simulink model "OFDM_Transceiver"  (R2013b)
settings: Solver=ode45  StartTime=0.0  StopTime=10.0  RelTol=1e-3
undefined symbols (not defined in the file or in its folder): A, N, xlipgetpartsetting
libraries: xbsIndex_r4 x35, commchan3 x2, commsink2 x2, commrandsrc2 x1, JTAGRuntimeCosim_r4 x1
settings Model: Creator=Lenovo  LastModifiedBy=Lenovo
settings OptimizationCC: ExpressionDepthLimit=2147483647
settings DebuggingCC: StateNameClashWarn=warning

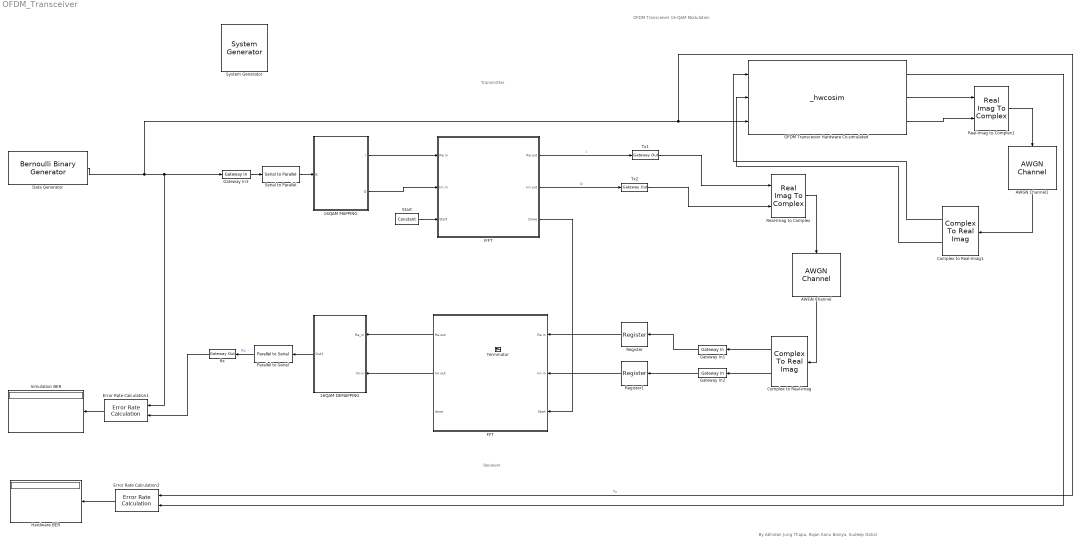
== system OFDM_Transceiver ==
  note: Transmitter
  note: Receiver
  note: OFDM Transceiver 16-QAM Modulation
  note: By Abhidan Jung Thapa, Rajan Kanu Baniya, Sudeep Dahal
  " System Generator" : xbsIndex_r4/ System Generator  Tag=genX  xilinxfamily=spartan3e  part=xc3s500e  speed=-4  package=fg320  synthesis_tool=XST  clock_wrapper=Clock Enables  directory=./netlist  proj_type=Project Navigator  Synth_file=XST Defaults  Impl_file=ISE Defaults  testbench=off  simulink_period=1  sysclk_period=20  dcm_input_clock_period=100  incr_netlist=off  trim_vbits=Everywhere in SubSystem  dbl_ovrd=According to Block Masks  core_generation=According to Block Masks  run_coregen=off  deprecated_control=off  eval_field=0  block_type=sysgen
      settings: block_version=10.1.3
  "16QAM DEMAPPING " : Subsystem
      mask Display: patch([0.363636 0.290909 0.4 0.290909 0.363636 0.490909 0.527273 0.563636 0.690909 0.581818 0.472727 0.4 0.509091 0.4 0.472727 0.581818 0.690909 0.563636 0.527273 0.490909 0.363636 ],[0.115385 0.269231 0.5 0.730769 0.884615 0.884615 0.807692 0.884615 0.884615 0.653846 0.884615 0.730769 0.5 0.269231 0.115385 0.346154 0.115385 0.115385 0.192308 0.115385 0.115385 ],[0.98 0.96 0.92]);
  16QAM MAPPING : Subsystem
      mask Display: patch([0.363636 0.290909 0.4 0.290909 0.363636 0.490909 0.527273 0.563636 0.690909 0.581818 0.472727 0.4 0.509091 0.4 0.472727 0.581818 0.690909 0.563636 0.527273 0.490909 0.363636 ],[0.115385 0.269231 0.5 0.730769 0.884615 0.884615 0.807692 0.884615 0.884615 0.653846 0.884615 0.730769 0.5 0.269231 0.115385 0.346154 0.115385 0.115385 0.192308 0.115385 0.115385 ],[0.98 0.96 0.92]);
  AWGN Channel : commchan3/AWGN Channel  InputProcessing=Inherited (this choice will be removed - see release notes)  seed=67  noiseMode="Signal to noise ratio  (SNR)"  EbNodB=10  EsNodB=40  SNRdB=20  bitsPerSym=2  Ps=1  Tsym=4e-6/80  variance=1
  AWGN Channel1 : commchan3/AWGN Channel  InputProcessing=Inherited (this choice will be removed - see release notes)  seed=67  noiseMode="Signal to noise ratio  (SNR)"  EbNodB=10  EsNodB=40  SNRdB=20  bitsPerSym=2  Ps=1  Tsym=4e-6/80  variance=1
  Complex to Real-Imag : ComplexToRealImag
  Complex to Real-Imag1 : ComplexToRealImag
  Data Generator : commrandsrc2/Bernoulli Binary Generator  P=0.5  seed=61  Ts=1  frameBased=off  sampPerFrame=1  orient=off  outDataType=double
  Error Rate Calculation1 : commsink2/Error Rate Calculation  N=1672  st_delay=700  cp_mode=Entire frame  subframe=[]  PMode=Port  WsName=ErrorVec  RsMode2=off  stop=off  numErr=100  maxBits=1e6
  Error Rate Calculation2 : commsink2/Error Rate Calculation  N=1672  st_delay=700  cp_mode=Entire frame  subframe=[]  PMode=Port  WsName=ErrorVec  RsMode2=off  stop=off  numErr=100  maxBits=1e6
  FFT : Subsystem
      mask Display: patch([0.363636 0.290909 0.4 0.290909 0.363636 0.490909 0.527273 0.563636 0.690909 0.581818 0.472727 0.4 0.509091 0.4 0.472727 0.581818 0.690909 0.563636 0.527273 0.490909 0.363636 ],[0.115385 0.269231 0.5 0.730769 0.884615 0.884615 0.807692 0.884615 0.884615 0.653846 0.884615 0.730769 0.5 0.269231 0.115385 0.346154 0.115385 0.115385 0.192308 0.115385 0.115385 ],[0.98 0.96 0.92]);
  Gateway In1 : xbsIndex_r4/Gateway In  gui_display_data_type=Fixed-point  arith_type="Signed  (2's comp)"  n_bits=16  bin_pt=15  preci_type=Single  exp_width=8  frac_width=24  quantization="Round  (unbiased: +/- Inf)"  overflow=Saturate  period=4  dbl_ovrd=off  timing_constraint=None  locs_specified=off  LOCs={}  UseAsADC=off  ADCChannel='1'  inherit_from_input=off  hdl_port=on  block_type=gatewayin
  Gateway In2 : xbsIndex_r4/Gateway In  gui_display_data_type=Fixed-point  arith_type="Signed  (2's comp)"  n_bits=16  bin_pt=15  preci_type=Single  exp_width=8  frac_width=24  quantization="Round  (unbiased: +/- Inf)"  overflow=Saturate  period=4  dbl_ovrd=off  timing_constraint=None  locs_specified=off  LOCs={}  UseAsADC=off  ADCChannel='1'  inherit_from_input=off  hdl_port=on  block_type=gatewayin
  Gateway In3 : xbsIndex_r4/Gateway In  gui_display_data_type=Fixed-point  arith_type=Unsigned  n_bits=1  bin_pt=0  preci_type=Single  exp_width=8  frac_width=24  quantization="Round  (unbiased: +/- Inf)"  overflow=Saturate  period=1  dbl_ovrd=off  timing_constraint=None  locs_specified=off  LOCs={}  UseAsADC=off  ADCChannel='1'  inherit_from_input=off  hdl_port=on  block_type=gatewayin
  Hardware BER : Display
  IFFT : Subsystem
      mask Display: patch([0.363636 0.290909 0.4 0.290909 0.363636 0.490909 0.527273 0.563636 0.690909 0.581818 0.472727 0.4 0.509091 0.4 0.472727 0.581818 0.690909 0.563636 0.527273 0.490909 0.363636 ],[0.115385 0.269231 0.5 0.730769 0.884615 0.884615 0.807692 0.884615 0.884615 0.653846 0.884615 0.730769 0.5 0.269231 0.115385 0.346154 0.115385 0.115385 0.192308 0.115385 0.115385 ],[0.98 0.96 0.92]);
  "OFDM Transceiver Hardware Co-simulated " : JTAGRuntimeCosim_r4/_hwcosim  clkSrc=Single Stepped  hasCombinationalPath=on  bitfileName=E:\FPGA\FinalYearProject\netlist\ofdm_final_october31_cw.bit  skipConfig=off  cable=Auto Detect  speed=N/A  cablePort=N/A  cableLocation=Local  shareCable=off  enable_codebug=on  design_xtable=|  engineDll=JTAGCosimEngine.dll  cableWaitTime=10  bscanPos=1  IRLengths=[6,8,8]  useWaitBox=1  hasBufgmux=on  Scheme=Cosim  useCmdProc=1  hasProc=0  useImpact=0  printLogFile=0  block_type=jtagcosim
      | {
      |   'clkWrapper' => 'ofdm_final_october31_cw',
      |   'clocksGcd' => undef,
      |   'device' => 'xc3s500e-4fg320',
      |   'ports' => {
      |     'gateway_in1' => {
      |       'bd_port_index' => 0,
      |       'direction' => 'in',
      |       'icon_text' => 'Gateway In1',
      |       'period' => 4,
      |       'sim_pause_trigger' => false,
      |       'type' => 'Fix_16_15',
      |       'width' => 16,
      |     },
      |     'gateway_in2' => {
      |       'bd_port_index' => 1,
      |       'direction' => 'in',
      |       'icon_text' => 'Gateway In2',
      |       'period' => 4,
      |       'sim_pause_trigger' => false,
      |       'type' => 'Fix_16_15',
      |       'width' => 16,
      |     },
      |     'gateway_in3' => {
      |       'bd_port_index' => 2,
      |       'direction' => 'in',
      |       'icon_text' => 'Gateway In3',
      |       'period' => 1,
      |       'sim_pause_trigger' => false,
      |       'type' => 'UFix_1_0',
      |       'width' => 1,
      |     },
      |     'rx' => {
      |       'bd_port_index' => 0,
      |       'direction' => 'out',
      |       'icon_text' => 'Rx',
      |       'period' => 1,
      |       'sim_pause_trigger' => false,
      |       'type' => 'UFix_1_0',
      |       'width' => 1,
      |     },
      |     'tx1' => {
      |       'bd_port_index' => 1,
      |       'direction' => 'out',
      |       'icon_text' => 'Tx1',
      |       'period' => 4,
      |       'sim_pause_trigger' => false,
      |       'type' => 'Fix_16_15',
      |       'width' => 16,
      |     },
      |     'tx2' => {
      |       'bd_port_index' => 2,
      |       'direction' => 'out',
      |       'icon_text' => 'Tx2',
      |       'period' => 4,
      |       'sim_pause_trigger' => false,
      |       'type' => 'Fix_16_15',
      |       'width' => 16,
      |     },
      |   },
      |   'shared_memories' => {},
      | }
  Parallel to Serial : xbsIndex_r4/Parallel to Serial  output_order=Least Significant Word First  arith_type=Unsigned  output_bits=1  bin_pt=0  rst=off  en=off  latency=0  dbl_ovrd=off  block_type=p2s
      settings: infoedit=Each sample presented at the input becomes several samples presented serially at the output.  xl_area=[4 5 0 4 0 0 0]  block_version=10.1.3
  Real-Imag to Complex : RealImagToComplex
  Real-Imag to Complex1 : RealImagToComplex
  Register : xbsIndex_r4/Register  init=0  rst=off  en=off  dbl_ovrd=off  block_type=register
  Register1 : xbsIndex_r4/Register  init=0  rst=off  en=off  dbl_ovrd=off  block_type=register
  Rx : xbsIndex_r4/Gateway Out  inherit_from_input=off  hdl_port=on  timing_constraint=None  locs_specified=off  LOCs={}  UseAsDAC=off  DACChannel='1'  block_type=gatewayout
      settings: infoedit="Gateway out block.  Converts Xilinx fixed point inputs into ouputs of type Simulink integer, double, or fixed point.<br><br>Hardware notes:  In hardware these blocks become top level output ports or are discarded, depending on how they are configured."  block_version=10.1.3
  Serial to Parallel : xbsIndex_r4/Serial to Parallel  input_order=Least Significant Word First  arith_type=Unsigned  output_bits=4  bin_pt=0  rst=off  en=off  latency=1  dbl_ovrd=off  block_type=s2p
      settings: infoedit=Groups of samples presented serially at the input become single samples presented at the output.  xl_area=[4 8 0 1 0 0 0]  block_version=10.1.3
  Simulation BER : Display
  Start : xbsIndex_r4/Constant  const=1  gui_display_data_type=Fixed-point  arith_type=Boolean  n_bits=16  bin_pt=14  preci_type=Single  exp_width=8  frac_width=24  explicit_period=off  period=1  equ=P=C  opselect=C  inp2=PCIN>>17  opr=+  inp1=P  carry=CIN  dbl_ovrd=off  block_type=constant
  Terminator : Terminator
  Tx1 : xbsIndex_r4/Gateway Out  inherit_from_input=off  hdl_port=on  timing_constraint=None  locs_specified=off  LOCs={}  UseAsDAC=off  DACChannel='1'  block_type=gatewayout
      settings: block_version=10.1.3
  Tx2 : xbsIndex_r4/Gateway Out  inherit_from_input=off  hdl_port=on  timing_constraint=None  locs_specified=off  LOCs={}  UseAsDAC=off  DACChannel='1'  block_type=gatewayout
      settings: block_version=10.1.3
  wires:
  Error Rate Calculation1/1 -> Simulation BER/1
  IFFT/3(Done) -> FFT/3(Start)
  Parallel to Serial/1 -> Rx/1  "Rx"
  Serial to Parallel/1 -> 16QAM MAPPING/1(B)
  Start/1 -> IFFT/3(Start)
  16QAM MAPPING/2(Q) -> IFFT/2(Im in)
  16QAM MAPPING/1(I) -> IFFT/1(Re in)
  Real-Imag to Complex/1 -> AWGN Channel/1
  IFFT/1(Re out) -> Tx1/1  "I"
  IFFT/2(Im out) -> Tx2/1  "Q"
  Complex to Real-Imag/1 -> Gateway In1/1
  Complex to Real-Imag/2 -> Gateway In2/1
  Gateway In1/1 -> Register/1
  Gateway In2/1 -> Register1/1
  Tx2/1 -> Real-Imag to Complex/2
  Tx1/1 -> Real-Imag to Complex/1
  Register1/1 -> FFT/2(Im in)
  AWGN Channel/1 -> Complex to Real-Imag/1
  Gateway In3/1 -> Serial to Parallel/1
  Data Generator/1 -> Gateway In3/1, Error Rate Calculation1/1, Error Rate Calculation2/1, "OFDM Transceiver Hardware Co-simulated "/3  "Tx"
  Error Rate Calculation2/1 -> Hardware BER/1
  FFT/1(Re out) -> "16QAM DEMAPPING "/1(Re_in)
  FFT/2(Im out) -> "16QAM DEMAPPING "/2(Im-in)
  "16QAM DEMAPPING "/1(Out1) -> Parallel to Serial/1
  Register/1 -> FFT/1(Re in)
  "OFDM Transceiver Hardware Co-simulated "/2 -> Real-Imag to Complex1/1
  "OFDM Transceiver Hardware Co-simulated "/3 -> Real-Imag to Complex1/2
  Real-Imag to Complex1/1 -> AWGN Channel1/1
  AWGN Channel1/1 -> Complex to Real-Imag1/1
  Complex to Real-Imag1/1 -> "OFDM Transceiver Hardware Co-simulated "/1
  Complex to Real-Imag1/2 -> "OFDM Transceiver Hardware Co-simulated "/2
  "OFDM Transceiver Hardware Co-simulated "/1 -> Error Rate Calculation2/2
  Rx/1 -> Error Rate Calculation1/2

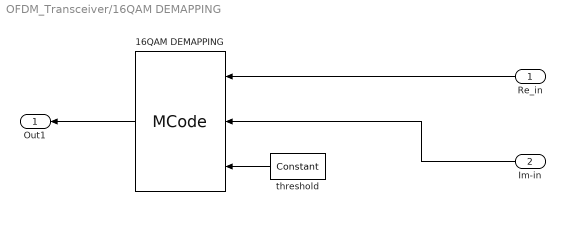
== system OFDM_Transceiver/16QAM DEMAPPING  ==
  Re_in : Inport
  Im-in : Inport  Port=2
  16QAM DEMAPPING : xbsIndex_r4/MCode  mfname=QAM16_DEM  explicit_period=off  period=1  inputsTable={'boundInpExpr'=>['','',''],'inputs'=>['I','Q','Thrd']}  outputsTable={'outputs'=>['B'],'suppressOut'=>['off']}  dbl_ovrd=off  enable_stdout=off  enable_debug=off  suppress_output=1  defparams={}  hide_port_list={}  block_type=mcode
      settings: xl_area=[60 0 0 110 0 0 0]  block_version=10.1.3
  threshold : xbsIndex_r4/Constant  const=0.25  gui_display_data_type=Fixed-point  arith_type=Signed (2's comp)  n_bits=16  bin_pt=15  preci_type=Single  exp_width=8  frac_width=24  explicit_period=off  period=1  equ=P=C  opselect=C  inp2=PCIN>>17  opr=+  inp1=P  carry=CIN  dbl_ovrd=off  block_type=constant
  Out1 : Outport
  wires:
  threshold/1 -> 16QAM DEMAPPING/3
  Im-in/1 -> 16QAM DEMAPPING/2
  16QAM DEMAPPING/1 -> Out1/1
  Re_in/1 -> 16QAM DEMAPPING/1

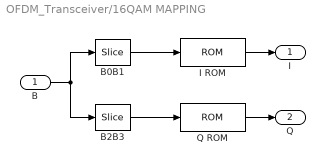
== system OFDM_Transceiver/16QAM MAPPING ==
  B : Inport
  B0B1 : xbsIndex_r4/Slice  nbits=2  boolean_output=off  mode=Lower Bit Location + Width  bit1=0  base1=LSB of Input  bit0=0  base0=LSB of Input  dbl_ovrd=off  block_type=slice
      settings: block_version=11.2
  B2B3 : xbsIndex_r4/Slice  nbits=2  boolean_output=off  mode=Upper Bit Location + Width  bit1=0  base1=MSB of Input  bit0=0  base0=MSB of Input  dbl_ovrd=off  block_type=slice
      settings: block_version=11.2
  I ROM : xbsIndex_r4/ROM  depth=4  initVector=[-3 +3 -1 +1]./3  distributed_mem=Block RAM  rst=off  init_reg=0  en=off  latency=1  gui_display_data_type=Fixed-point  arith_type="Signed  (2's comp)"  n_bits=16  bin_pt=15  preci_type=Single  exp_width=8  frac_width=24  dbl_ovrd=off  optimize=Area  use_rpm=on  block_type=sprom
      settings: xl_area=[0 0 1 0 0 0 0]  block_version=10.1.3
  Q ROM : xbsIndex_r4/ROM  depth=4  initVector=[-3 +3 -1 +1]./3  distributed_mem=Block RAM  rst=off  init_reg=0  en=off  latency=1  gui_display_data_type=Fixed-point  arith_type="Signed  (2's comp)"  n_bits=16  bin_pt=15  preci_type=Single  exp_width=8  frac_width=24  dbl_ovrd=off  optimize=Area  use_rpm=on  block_type=sprom
      settings: xl_area=[0 0 1 0 0 0 0]  block_version=10.1.3
  I : Outport
  Q : Outport  Port=2
  wires:
  B/1 -> B2B3/1, B0B1/1
  I ROM/1 -> I/1
  Q ROM/1 -> Q/1
  B0B1/1 -> I ROM/1
  B2B3/1 -> Q ROM/1

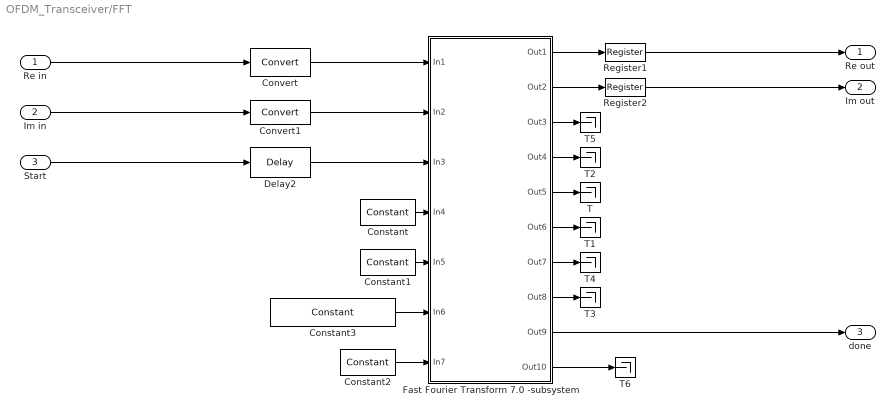
== system OFDM_Transceiver/FFT ==
  Re in : Inport
  Im in : Inport  Port=2
  Start : Inport  Port=3
  Constant : xbsIndex_r4/Constant  const=1  gui_display_data_type=Fixed-point  arith_type=Boolean  n_bits=16  bin_pt=14  preci_type=Single  exp_width=8  frac_width=24  explicit_period=off  period=1  equ=P=C  opselect=C  inp2=PCIN>>17  opr=+  inp1=P  carry=CIN  dbl_ovrd=off  block_type=constant
  Constant1 : xbsIndex_r4/Constant  const=1  gui_display_data_type=Fixed-point  arith_type=Boolean  n_bits=16  bin_pt=14  preci_type=Single  exp_width=8  frac_width=24  explicit_period=off  period=1  equ=P=C  opselect=C  inp2=PCIN>>17  opr=+  inp1=P  carry=CIN  dbl_ovrd=off  block_type=constant
  Constant2 : xbsIndex_r4/Constant  const=1  gui_display_data_type=Fixed-point  arith_type=Boolean  n_bits=16  bin_pt=14  preci_type=Single  exp_width=8  frac_width=24  explicit_period=off  period=1  equ=P=C  opselect=C  inp2=PCIN>>17  opr=+  inp1=P  carry=CIN  dbl_ovrd=off  block_type=constant
  Constant3 : xbsIndex_r4/Constant  const=bin2dec('00001')  gui_display_data_type=Fixed-point  arith_type=Unsigned  n_bits=6  bin_pt=0  preci_type=Single  exp_width=8  frac_width=24  explicit_period=off  period=1  equ=P=C  opselect=C  inp2=PCIN>>17  opr=+  inp1=P  carry=CIN  dbl_ovrd=off  block_type=constant
  Convert : xbsIndex_r4/Convert  gui_display_data_type=Fixed-point  arith_type="Signed  (2's comp)"  n_bits=16  bin_pt=15  float_type=Single  exp_bits=8  fraction_bits=24  quantization=Truncate  overflow=Wrap  en=off  latency=1  dbl_ovrd=off  pipeline=off  block_type=convert
      settings: xl_area=[0 16 0 0 0 0 0]  block_version=9.1
  Convert1 : xbsIndex_r4/Convert  gui_display_data_type=Fixed-point  arith_type="Signed  (2's comp)"  n_bits=16  bin_pt=15  float_type=Single  exp_bits=8  fraction_bits=24  quantization=Truncate  overflow=Wrap  en=off  latency=1  dbl_ovrd=off  pipeline=off  block_type=convert
      settings: xl_area=[0 16 0 0 0 0 0]  block_version=9.1
  Delay2 : xbsIndex_r4/Delay  rst=off  infoeditControl=Selection of Reset will increase slice count due to use of real FFs and instead of SRLs  en=off  latency=2  dbl_ovrd=off  reg_retiming=off  block_type=delay
      settings: xl_area=[1 1 0 1 0 0 0]
  Fast Fourier Transform 7.0 -subsystem : Subsystem
  Register1 : xbsIndex_r4/Register  init=0  rst=off  en=off  dbl_ovrd=off  block_type=register
      settings: xl_area=[8 16 0 0 0 0 0]  block_version=9.1
  Register2 : xbsIndex_r4/Register  init=0  rst=off  en=off  dbl_ovrd=off  block_type=register
      settings: xl_area=[8 16 0 0 0 0 0]  block_version=9.1
  T{,1..6} (7 alike) : Terminator
  Re out : Outport
  Im out : Outport  Port=2
  done : Outport  Port=3
  wires:
  Start/1 -> Delay2/1
  Im in/1 -> Convert1/1
  Register2/1 -> Im out/1
  Re in/1 -> Convert/1
  Register1/1 -> Re out/1
  Convert/1 -> Fast Fourier Transform 7.0 -subsystem/1(In1)
  Convert1/1 -> Fast Fourier Transform 7.0 -subsystem/2(In2)
  Delay2/1 -> Fast Fourier Transform 7.0 -subsystem/3(In3)
  Constant/1 -> Fast Fourier Transform 7.0 -subsystem/4(In4)
  Constant1/1 -> Fast Fourier Transform 7.0 -subsystem/5(In5)
  Constant3/1 -> Fast Fourier Transform 7.0 -subsystem/6(In6)
  Constant2/1 -> Fast Fourier Transform 7.0 -subsystem/7(In7)
  Fast Fourier Transform 7.0 -subsystem/1(Out1) -> Register1/1
  Fast Fourier Transform 7.0 -subsystem/2(Out2) -> Register2/1
  Fast Fourier Transform 7.0 -subsystem/3(Out3) -> T5/1
  Fast Fourier Transform 7.0 -subsystem/4(Out4) -> T2/1
  Fast Fourier Transform 7.0 -subsystem/5(Out5) -> T/1
  Fast Fourier Transform 7.0 -subsystem/6(Out6) -> T1/1
  Fast Fourier Transform 7.0 -subsystem/7(Out7) -> T4/1
  Fast Fourier Transform 7.0 -subsystem/8(Out8) -> T3/1
  Fast Fourier Transform 7.0 -subsystem/9(Out9) -> done/1
  Fast Fourier Transform 7.0 -subsystem/10(Out10) -> T6/1

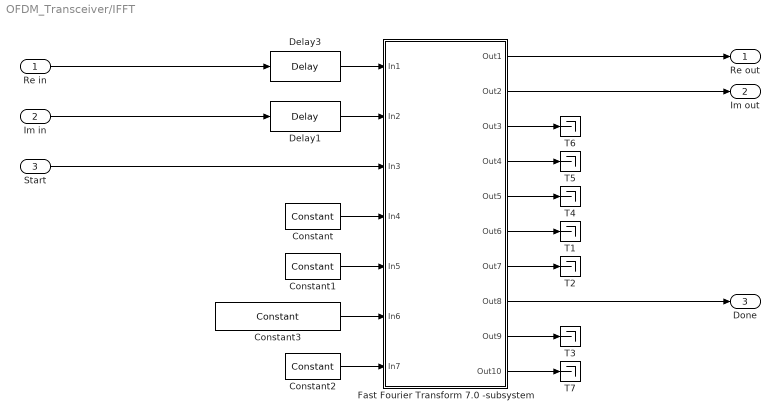
== system OFDM_Transceiver/IFFT ==
  Re in : Inport
  Im in : Inport  Port=2
  Start : Inport  Port=3
  Constant : xbsIndex_r4/Constant  const=0  gui_display_data_type=Fixed-point  arith_type=Boolean  n_bits=16  bin_pt=14  preci_type=Single  exp_width=8  frac_width=24  explicit_period=off  period=1  equ=P=C  opselect=C  inp2=PCIN>>17  opr=+  inp1=P  carry=CIN  dbl_ovrd=off  block_type=constant
  Constant1 : xbsIndex_r4/Constant  const=1  gui_display_data_type=Fixed-point  arith_type=Boolean  n_bits=16  bin_pt=14  preci_type=Single  exp_width=8  frac_width=24  explicit_period=off  period=1  equ=P=C  opselect=C  inp2=PCIN>>17  opr=+  inp1=P  carry=CIN  dbl_ovrd=off  block_type=constant
  Constant2 : xbsIndex_r4/Constant  const=1  gui_display_data_type=Fixed-point  arith_type=Boolean  n_bits=16  bin_pt=14  preci_type=Single  exp_width=8  frac_width=24  explicit_period=off  period=1  equ=P=C  opselect=C  inp2=PCIN>>17  opr=+  inp1=P  carry=CIN  dbl_ovrd=off  block_type=constant
  Constant3 : xbsIndex_r4/Constant  const=bin2dec('001111')  gui_display_data_type=Fixed-point  arith_type=Unsigned  n_bits=6  bin_pt=0  preci_type=Single  exp_width=8  frac_width=24  explicit_period=off  period=1  equ=P=C  opselect=C  inp2=PCIN>>17  opr=+  inp1=P  carry=CIN  dbl_ovrd=off  block_type=constant
  Delay1 : xbsIndex_r4/Delay  rst=off  infoeditControl=Selection of Reset will increase slice count due to use of real FFs and instead of SRLs  en=off  latency=1  dbl_ovrd=off  reg_retiming=off  block_type=delay
      settings: xl_area=[8 16 0 0 0 0 0]
  Delay3 : xbsIndex_r4/Delay  rst=off  infoeditControl=Selection of Reset will increase slice count due to use of real FFs and instead of SRLs  en=off  latency=1  dbl_ovrd=off  reg_retiming=off  block_type=delay
      settings: xl_area=[8 16 0 0 0 0 0]
  Fast Fourier Transform 7.0 -subsystem : Subsystem
  T{1..7} (7 alike) : Terminator
  Re out : Outport
  Im out : Outport  Port=2
  Done : Outport  Port=3
  wires:
  Im in/1 -> Delay1/1
  Re in/1 -> Delay3/1
  Delay3/1 -> Fast Fourier Transform 7.0 -subsystem/1(In1)
  Delay1/1 -> Fast Fourier Transform 7.0 -subsystem/2(In2)
  Start/1 -> Fast Fourier Transform 7.0 -subsystem/3(In3)
  Constant/1 -> Fast Fourier Transform 7.0 -subsystem/4(In4)
  Constant1/1 -> Fast Fourier Transform 7.0 -subsystem/5(In5)
  Constant3/1 -> Fast Fourier Transform 7.0 -subsystem/6(In6)
  Constant2/1 -> Fast Fourier Transform 7.0 -subsystem/7(In7)
  Fast Fourier Transform 7.0 -subsystem/1(Out1) -> Re out/1
  Fast Fourier Transform 7.0 -subsystem/2(Out2) -> Im out/1
  Fast Fourier Transform 7.0 -subsystem/3(Out3) -> T6/1
  Fast Fourier Transform 7.0 -subsystem/4(Out4) -> T5/1
  Fast Fourier Transform 7.0 -subsystem/5(Out5) -> T4/1
  Fast Fourier Transform 7.0 -subsystem/6(Out6) -> T1/1
  Fast Fourier Transform 7.0 -subsystem/7(Out7) -> T2/1
  Fast Fourier Transform 7.0 -subsystem/8(Out8) -> Done/1
  Fast Fourier Transform 7.0 -subsystem/9(Out9) -> T3/1
  Fast Fourier Transform 7.0 -subsystem/10(Out10) -> T7/1

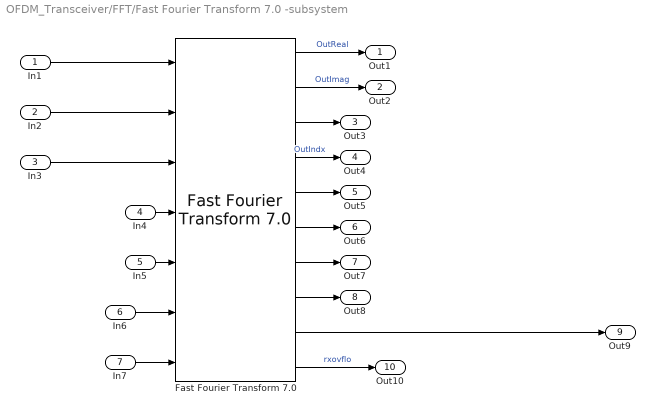
== system OFDM_Transceiver/FFT/Fast Fourier Transform 7.0 -subsystem ==
  In1 : Inport
  In2 : Inport  Port=2
  In3 : Inport  Port=3
  In4 : Inport  Port=4
  In5 : Inport  Port=5
  In6 : Inport  Port=6
  In7 : Inport  Port=7
  "Fast Fourier Transform 7.0 " : xbsIndex_r4/Fast Fourier Transform 7.0   transform_length=64  implementation_options=automatically_select  target_clock_frequency=50  target_data_throughput=50  run_time_configurable_transform_length=off  phase_factor_width=16  scaling_options=scaled  rounding_modes=truncation  output_ordering=natural_order  cyclic_prefix_insertion=off  ce=off  sclr=off  ovflo=on  input_data_offset=no_offset  memory_options_data=block_ram  memory_options_phase_factors=block_ram  number_of_stages_using_block_ram_for_data_and_phase_factors=0  memory_options_reorder=distributed_ram  memory_options_hybrid=off  complex_mult_type=use_mults_resources  butterfly_type=use_luts  channels=1  input_ordering=natural_order  input_width=16  simulation_type=external_xfix  simulation_model=fftv7_CModel:fftv7_cmodel  ip_name=Fast Fourier Transform  ip_version=7.0  dsptool_ready=true  wrapper_available=true  port_translation_map={ 'ce' => 'en', 'sclr' => 'rst' }  ipcore_fpga_part=xlipgetpartsetting(gcb, {'virtex4', 'xc4vsx35', '-10', 'ff668'})  block_type=xfft_v7_0
      settings: xl_area=[1127 1579 1 1572 0 22 0]  block_version=11.2
  Out1 : Outport
  Out2 : Outport  Port=2
  Out3 : Outport  Port=3
  Out4 : Outport  Port=4
  Out5 : Outport  Port=5
  Out6 : Outport  Port=6
  Out7 : Outport  Port=7
  Out8 : Outport  Port=8
  Out9 : Outport  Port=9
  Out10 : Outport  Port=10
  wires:
  "Fast Fourier Transform 7.0 "/9 -> Out9/1
  "Fast Fourier Transform 7.0 "/7 -> Out7/1
  In3/1 -> "Fast Fourier Transform 7.0 "/3
  "Fast Fourier Transform 7.0 "/6 -> Out6/1
  In5/1 -> "Fast Fourier Transform 7.0 "/5
  In4/1 -> "Fast Fourier Transform 7.0 "/4
  In1/1 -> "Fast Fourier Transform 7.0 "/1
  In2/1 -> "Fast Fourier Transform 7.0 "/2
  "Fast Fourier Transform 7.0 "/8 -> Out8/1
  "Fast Fourier Transform 7.0 "/3 -> Out3/1
  "Fast Fourier Transform 7.0 "/10 -> Out10/1  "rxovflo"
  "Fast Fourier Transform 7.0 "/2 -> Out2/1  "OutImag"
  In7/1 -> "Fast Fourier Transform 7.0 "/7
  "Fast Fourier Transform 7.0 "/1 -> Out1/1  "OutReal"
  In6/1 -> "Fast Fourier Transform 7.0 "/6
  "Fast Fourier Transform 7.0 "/5 -> Out5/1
  "Fast Fourier Transform 7.0 "/4 -> Out4/1  "OutIndx"

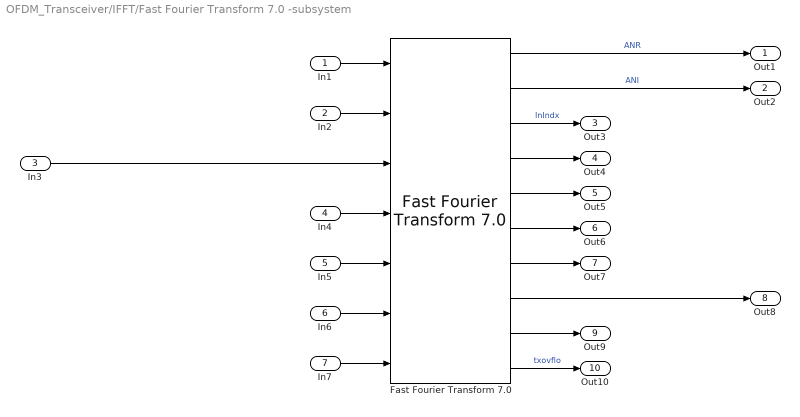
== system OFDM_Transceiver/IFFT/Fast Fourier Transform 7.0 -subsystem ==
  In1 : Inport
  In2 : Inport  Port=2
  In3 : Inport  Port=3
  In4 : Inport  Port=4
  In5 : Inport  Port=5
  In6 : Inport  Port=6
  In7 : Inport  Port=7
  "Fast Fourier Transform 7.0 " : xbsIndex_r4/Fast Fourier Transform 7.0   transform_length=64  implementation_options=automatically_select  target_clock_frequency=50  target_data_throughput=50  run_time_configurable_transform_length=off  phase_factor_width=16  scaling_options=scaled  rounding_modes=truncation  output_ordering=natural_order  cyclic_prefix_insertion=off  ce=off  sclr=off  ovflo=on  input_data_offset=no_offset  memory_options_data=block_ram  memory_options_phase_factors=block_ram  number_of_stages_using_block_ram_for_data_and_phase_factors=0  memory_options_reorder=distributed_ram  memory_options_hybrid=off  complex_mult_type=use_mults_resources  butterfly_type=use_luts  channels=1  input_ordering=natural_order  input_width=16  simulation_type=external_xfix  simulation_model=fftv7_CModel:fftv7_cmodel  ip_name=Fast Fourier Transform  ip_version=7.0  dsptool_ready=true  wrapper_available=true  port_translation_map={ 'ce' => 'en', 'sclr' => 'rst' }  ipcore_fpga_part=xlipgetpartsetting(gcb, {'virtex4', 'xc4vsx35', '-10', 'ff668'})  block_type=xfft_v7_0
      settings: xl_area=[1127 1579 1 1572 0 22 0]  block_version=11.2
  Out1 : Outport
  Out2 : Outport  Port=2
  Out3 : Outport  Port=3
  Out4 : Outport  Port=4
  Out5 : Outport  Port=5
  Out6 : Outport  Port=6
  Out7 : Outport  Port=7
  Out8 : Outport  Port=8
  Out9 : Outport  Port=9
  Out10 : Outport  Port=10
  wires:
  "Fast Fourier Transform 7.0 "/1 -> Out1/1  "ANR"
  In4/1 -> "Fast Fourier Transform 7.0 "/4
  In5/1 -> "Fast Fourier Transform 7.0 "/5
  "Fast Fourier Transform 7.0 "/3 -> Out3/1  "InIndx"
  In1/1 -> "Fast Fourier Transform 7.0 "/1
  "Fast Fourier Transform 7.0 "/6 -> Out6/1
  In2/1 -> "Fast Fourier Transform 7.0 "/2
  In3/1 -> "Fast Fourier Transform 7.0 "/3
  "Fast Fourier Transform 7.0 "/4 -> Out4/1
  "Fast Fourier Transform 7.0 "/9 -> Out9/1
  "Fast Fourier Transform 7.0 "/2 -> Out2/1  "ANI"
  "Fast Fourier Transform 7.0 "/7 -> Out7/1
  "Fast Fourier Transform 7.0 "/8 -> Out8/1
  "Fast Fourier Transform 7.0 "/10 -> Out10/1  "txovflo"
  In7/1 -> "Fast Fourier Transform 7.0 "/7
  In6/1 -> "Fast Fourier Transform 7.0 "/6
  "Fast Fourier Transform 7.0 "/5 -> Out5/1
